simulink model "MIL4L3_SW6_V1_20220211"  (R2018b)
settings: Solver=FixedStepAuto  StartTime=0.0  StopTime=inf  FixedStep=0.001  RelTol=1e-3
PreLoadFcn:
  | A0_MILtest;
undefined symbols (not defined in the file or in its folder): Clb_ICADirect_LaneDisp_StateFive, Clb_ICADirect_LaneDisp_StateFour, Clb_ICADirect_LaneDisp_StateOne, Clb_ICADirect_LaneDisp_StateThree, Clb_ICADirect_LaneDisp_StateTwo, Clb_ICADirect_LaneDisp_StateZero, Clb_ICADirect_LaneDispSW, Clb_ICADirect_TrnLghtsCom_Switch, Clb_ICADirect_TrnLghtsCom_Value, Clb_ICADirect_TrnLghtsCrtl_Inhb, IMAP_Clb_ACU_Driver_Belt, IMAP_Clb_ACU_Driver_Belt_Over, IMAP_Clb_ACU_Passenger_Belt, IMAP_Clb_ACU_Passenger_Belt_Over, IMAP_Clb_ACU_RearLeft_Belt, IMAP_Clb_ACU_RearLeft_Belt_Over, IMAP_Clb_ACU_RearMiddle_Belt, IMAP_Clb_ACU_RearMiddle_Belt_Over, IMAP_Clb_ACU_RearRight_Belt, IMAP_Clb_ACU_RearRight_Belt_Over, IMAP_Clb_AEB_Switch, IMAP_Clb_AEB_Switch_Over, IMAP_Clb_ALC_TLC_Mode, IMAP_Clb_ALC_TLC_Mode_Over, IMAP_Clb_BCM_Battery_Voltage, IMAP_Clb_BCM_Battery_Voltage_Over, IMAP_Clb_BCM_BrakeLamp_State, IMAP_Clb_BCM_BrakeLamp_State_Over, IMAP_Clb_BCM_CHMSL_Status, IMAP_Clb_BCM_CHMSL_Status_Over, IMAP_Clb_BCM_Door_Lock_State, IMAP_Clb_BCM_Door_Lock_State_Over, IMAP_Clb_BCM_FrontWiper_State, IMAP_Clb_BCM_FrontWiper_State_Over, IMAP_Clb_BCM_FrontWiper_Switch, IMAP_Clb_BCM_FrontWiper_Switch_Over, IMAP_Clb_BCM_HazardLamp, IMAP_Clb_BCM_HazardLamp_Over, IMAP_Clb_BCM_HazardLamp_Switch, IMAP_Clb_BCM_HazardLamp_Switch_Over, IMAP_Clb_BCM_HighBeam_State, IMAP_Clb_BCM_HighBeam_State_Over, IMAP_Clb_BCM_Ignition_State, IMAP_Clb_BCM_Ignition_State_Over, IMAP_Clb_BCM_IHBC_Enabled, IMAP_Clb_BCM_IHBC_Enabled_Over, IMAP_Clb_BCM_Left_Light, IMAP_Clb_BCM_Left_Light_Over, IMAP_Clb_BCM_LeftTurn_Switch, IMAP_Clb_BCM_LeftTurn_Switch_Over, IMAP_Clb_BCM_LF_Door_State, IMAP_Clb_BCM_LF_Door_State_Over, IMAP_Clb_BCM_LowBeam_State, IMAP_Clb_BCM_LowBeam_State_Over, IMAP_Clb_BCM_LR_Door_State, IMAP_Clb_BCM_LR_Door_State_Over, IMAP_Clb_BCM_RF_Door_State, IMAP_Clb_BCM_RF_Door_State_Over, IMAP_Clb_BCM_Right_Light, IMAP_Clb_BCM_Right_Light_Over ... (+547)
libraries: CarMaker4SL x2153, simulink x292, dspstat3 x3, canmsglib x2, simulink_extras x1
(part 29 of 52)

== system MIL4L3_SW6_V1_20220211/CarMaker/VehicleControl/Data Inport/IMAP/Subsystem18/Subsystem5 ==
  In1 : Inport
  -1 : Constant
  -2 : Constant
  -3 : Constant  Value=13.515
  -4 : Constant
  0 : Constant
  1 : Constant  Value=15.604
  2 : Constant  Value=11.1
  3 : Constant  Value=6.986
  4 : Constant  Value=4.737
  5 : Constant  Value=3.311
  6 : Constant  Value=2.356
  Multiport Switch : MultiPortSwitch  DataPortOrder=Specify indices  Inputs=9  DataPortIndices={0,1,2,3,4,5,6,7,8,-1}  DataPortForDefault=Additional data port
  TCU_AGB_position : Outport
  wires:
  -4/1 -> Multiport Switch/12
  -3/1 -> Multiport Switch/11
  Multiport Switch/1 -> TCU_AGB_position/1  "TCU_AGB_position"
  -2/1 -> Multiport Switch/10
  6/1 -> Multiport Switch/8
  1/1 -> Multiport Switch/3
  5/1 -> Multiport Switch/7
  In1/1 -> Multiport Switch/1
  2/1 -> Multiport Switch/4
  0/1 -> Multiport Switch/2
  -1/1 -> Multiport Switch/9
  4/1 -> Multiport Switch/6
  3/1 -> Multiport Switch/5

== system MIL4L3_SW6_V1_20220211/CarMaker/VehicleControl/Data Inport/SDFA-L3/Subsystem4/Subsystem ==
  Constant4 : Constant  Value=0
  Digital Clock : DigitalClock  SampleTime=0.055
  Gain9 : Gain  Gain=100/5.5
  Switch : Switch  Threshold=65535
  Out1 : Outport
  wires:
  Digital Clock/1 -> Gain9/1
  Constant4/1 -> Switch/1
  Switch/1 -> Out1/1
  Gain9/1 -> Switch/2, Switch/3

== system MIL4L3_SW6_V1_20220211/CarMaker/VehicleControl/Data Inport/SDFA-L3/Subsystem4/Subsystem1 ==
  Constant4 : Constant  Value=0
  Digital Clock : DigitalClock  SampleTime=0.055
  Gain9 : Gain  Gain=100/5.5
  Switch : Switch  Threshold=65535
  Out1 : Outport
  wires:
  Gain9/1 -> Switch/3, Switch/2
  Switch/1 -> Out1/1
  Constant4/1 -> Switch/1
  Digital Clock/1 -> Gain9/1

== system MIL4L3_SW6_V1_20220211/CarMaker/VehicleControl/Data Inport/SDFA-L3/Subsystem4/Subsystem10 ==
  Constant4 : Constant  Value=0
  Digital Clock : DigitalClock  SampleTime=0.055
  Gain9 : Gain  Gain=100/5.5
  Switch : Switch  Threshold=65535
  Out1 : Outport
  wires:
  Digital Clock/1 -> Gain9/1
  Constant4/1 -> Switch/1
  Switch/1 -> Out1/1
  Gain9/1 -> Switch/2, Switch/3

== system MIL4L3_SW6_V1_20220211/CarMaker/VehicleControl/Data Inport/SDFA-L3/Subsystem4/Subsystem11 ==
  Constant4 : Constant  Value=0
  Digital Clock : DigitalClock  SampleTime=0.055
  Gain9 : Gain  Gain=100/5.5
  Switch : Switch  Threshold=65535
  Out1 : Outport
  wires:
  Gain9/1 -> Switch/3, Switch/2
  Switch/1 -> Out1/1
  Constant4/1 -> Switch/1
  Digital Clock/1 -> Gain9/1

== system MIL4L3_SW6_V1_20220211/CarMaker/VehicleControl/Data Inport/SDFA-L3/Subsystem4/Subsystem12 ==
  Constant4 : Constant  Value=0
  Digital Clock : DigitalClock  SampleTime=0.055
  Gain9 : Gain  Gain=100/5.5
  Switch : Switch  Threshold=65535
  Out1 : Outport
  wires:
  Digital Clock/1 -> Gain9/1
  Constant4/1 -> Switch/1
  Switch/1 -> Out1/1
  Gain9/1 -> Switch/2, Switch/3

== system MIL4L3_SW6_V1_20220211/CarMaker/VehicleControl/Data Inport/SDFA-L3/Subsystem4/Subsystem13 ==
  Constant4 : Constant  Value=0
  Digital Clock : DigitalClock  SampleTime=0.055
  Gain9 : Gain  Gain=100/5.5
  Switch : Switch  Threshold=65535
  Out1 : Outport
  wires:
  Gain9/1 -> Switch/3, Switch/2
  Switch/1 -> Out1/1
  Constant4/1 -> Switch/1
  Digital Clock/1 -> Gain9/1

== system MIL4L3_SW6_V1_20220211/CarMaker/VehicleControl/Data Inport/SDFA-L3/Subsystem4/Subsystem14 ==
  Constant4 : Constant  Value=0
  Digital Clock : DigitalClock  SampleTime=0.055
  Gain9 : Gain  Gain=100/5.5
  Switch : Switch  Threshold=65535
  Out1 : Outport
  wires:
  Gain9/1 -> Switch/3, Switch/2
  Switch/1 -> Out1/1
  Constant4/1 -> Switch/1
  Digital Clock/1 -> Gain9/1

== system MIL4L3_SW6_V1_20220211/CarMaker/VehicleControl/Data Inport/SDFA-L3/Subsystem4/Subsystem15 ==
  Constant4 : Constant  Value=0
  Digital Clock : DigitalClock  SampleTime=0.055
  Gain9 : Gain  Gain=100/5.5
  Switch : Switch  Threshold=65535
  Out1 : Outport
  wires:
  Digital Clock/1 -> Gain9/1
  Constant4/1 -> Switch/1
  Switch/1 -> Out1/1
  Gain9/1 -> Switch/2, Switch/3

== system MIL4L3_SW6_V1_20220211/CarMaker/VehicleControl/Data Inport/SDFA-L3/Subsystem4/Subsystem16 ==
  Constant4 : Constant  Value=0
  Digital Clock : DigitalClock  SampleTime=0.055
  Gain9 : Gain  Gain=100/5.5
  Switch : Switch  Threshold=65535
  Out1 : Outport
  wires:
  Gain9/1 -> Switch/3, Switch/2
  Switch/1 -> Out1/1
  Constant4/1 -> Switch/1
  Digital Clock/1 -> Gain9/1

== system MIL4L3_SW6_V1_20220211/CarMaker/VehicleControl/Data Inport/SDFA-L3/Subsystem4/Subsystem17 ==
  Constant4 : Constant  Value=0
  Digital Clock : DigitalClock  SampleTime=0.055
  Gain9 : Gain  Gain=100/5.5
  Switch : Switch  Threshold=65535
  Out1 : Outport
  wires:
  Digital Clock/1 -> Gain9/1
  Constant4/1 -> Switch/1
  Switch/1 -> Out1/1
  Gain9/1 -> Switch/2, Switch/3

== system MIL4L3_SW6_V1_20220211/CarMaker/VehicleControl/Data Inport/SDFA-L3/Subsystem4/Subsystem18 ==
  Constant4 : Constant  Value=0
  Digital Clock : DigitalClock  SampleTime=0.055
  Gain9 : Gain  Gain=100/5.5
  Switch : Switch  Threshold=65535
  Out1 : Outport
  wires:
  Digital Clock/1 -> Gain9/1
  Constant4/1 -> Switch/1
  Switch/1 -> Out1/1
  Gain9/1 -> Switch/2, Switch/3

== system MIL4L3_SW6_V1_20220211/CarMaker/VehicleControl/Data Inport/SDFA-L3/Subsystem4/Subsystem19 ==
  Constant4 : Constant  Value=0
  Digital Clock : DigitalClock  SampleTime=0.055
  Gain9 : Gain  Gain=100/5.5
  Switch : Switch  Threshold=65535
  Out1 : Outport
  wires:
  Gain9/1 -> Switch/3, Switch/2
  Switch/1 -> Out1/1
  Constant4/1 -> Switch/1
  Digital Clock/1 -> Gain9/1

== system MIL4L3_SW6_V1_20220211/CarMaker/VehicleControl/Data Inport/SDFA-L3/Subsystem4/Subsystem2 ==
  Constant4 : Constant  Value=0
  Digital Clock : DigitalClock  SampleTime=0.055
  Gain9 : Gain  Gain=100/5.5
  Switch : Switch  Threshold=65535
  Out1 : Outport
  wires:
  Gain9/1 -> Switch/3, Switch/2
  Switch/1 -> Out1/1
  Constant4/1 -> Switch/1
  Digital Clock/1 -> Gain9/1

== system MIL4L3_SW6_V1_20220211/CarMaker/VehicleControl/Data Inport/SDFA-L3/Subsystem4/Subsystem3 ==
  Constant4 : Constant  Value=0
  Digital Clock : DigitalClock  SampleTime=0.055
  Gain9 : Gain  Gain=100/5.5
  Switch : Switch  Threshold=65535
  Out1 : Outport
  wires:
  Digital Clock/1 -> Gain9/1
  Constant4/1 -> Switch/1
  Switch/1 -> Out1/1
  Gain9/1 -> Switch/2, Switch/3

== system MIL4L3_SW6_V1_20220211/CarMaker/VehicleControl/Data Inport/SDFA-L3/Subsystem4/Subsystem4 ==
  Constant4 : Constant  Value=0
  Digital Clock : DigitalClock  SampleTime=0.055
  Gain9 : Gain  Gain=100/5.5
  Switch : Switch  Threshold=65535
  Out1 : Outport
  wires:
  Gain9/1 -> Switch/3, Switch/2
  Switch/1 -> Out1/1
  Constant4/1 -> Switch/1
  Digital Clock/1 -> Gain9/1

== system MIL4L3_SW6_V1_20220211/CarMaker/VehicleControl/Data Inport/SDFA-L3/Subsystem4/Subsystem5 ==
  Constant4 : Constant  Value=0
  Digital Clock : DigitalClock  SampleTime=0.055
  Gain9 : Gain  Gain=100/5.5
  Switch : Switch  Threshold=65535
  Out1 : Outport
  wires:
  Digital Clock/1 -> Gain9/1
  Constant4/1 -> Switch/1
  Switch/1 -> Out1/1
  Gain9/1 -> Switch/2, Switch/3

== system MIL4L3_SW6_V1_20220211/CarMaker/VehicleControl/Data Inport/SDFA-L3/Subsystem4/Subsystem6 ==
  Constant4 : Constant  Value=0
  Digital Clock : DigitalClock  SampleTime=0.055
  Gain9 : Gain  Gain=100/5.5
  Switch : Switch  Threshold=65535
  Out1 : Outport
  wires:
  Digital Clock/1 -> Gain9/1
  Constant4/1 -> Switch/1
  Switch/1 -> Out1/1
  Gain9/1 -> Switch/2, Switch/3

== system MIL4L3_SW6_V1_20220211/CarMaker/VehicleControl/Data Inport/SDFA-L3/Subsystem4/Subsystem7 ==
  Constant4 : Constant  Value=0
  Digital Clock : DigitalClock  SampleTime=0.055
  Gain9 : Gain  Gain=100/5.5
  Switch : Switch  Threshold=65535
  Out1 : Outport
  wires:
  Gain9/1 -> Switch/3, Switch/2
  Switch/1 -> Out1/1
  Constant4/1 -> Switch/1
  Digital Clock/1 -> Gain9/1

== system MIL4L3_SW6_V1_20220211/CarMaker/VehicleControl/Data Inport/SDFA-L3/Subsystem4/Subsystem8 ==
  Constant4 : Constant  Value=0
  Digital Clock : DigitalClock  SampleTime=0.055
  Gain9 : Gain  Gain=100/5.5
  Switch : Switch  Threshold=65535
  Out1 : Outport
  wires:
  Gain9/1 -> Switch/3, Switch/2
  Switch/1 -> Out1/1
  Constant4/1 -> Switch/1
  Digital Clock/1 -> Gain9/1

== system MIL4L3_SW6_V1_20220211/CarMaker/VehicleControl/Data Inport/SDFA-L3/Subsystem4/Subsystem9 ==
  Constant4 : Constant  Value=0
  Digital Clock : DigitalClock  SampleTime=0.055
  Gain9 : Gain  Gain=100/5.5
  Switch : Switch  Threshold=65535
  Out1 : Outport
  wires:
  Digital Clock/1 -> Gain9/1
  Constant4/1 -> Switch/1
  Switch/1 -> Out1/1
  Gain9/1 -> Switch/2, Switch/3

== system MIL4L3_SW6_V1_20220211/CarMaker/VehicleControl/Data Inport/SDFA-L3/Subsystem40/Subsystem ==
  Compare To Constant : simulink/Logic and Bit Operations/Compare To Constant  relop=>=  const=1  OutDataTypeStr=boolean
  Compare To Constant1 : simulink/Logic and Bit Operations/Compare To Constant  relop=>  const=0  OutDataTypeStr=boolean
  Const tar_id5 : Constant  Value=0
  Data Type Conversion : DataTypeConversion
  Digital Clock : DigitalClock  SampleTime=0.06
  Logical Operator : Logic  AllPortsSameDT=off  OutDataTypeStr=boolean
  Read CM Dict1 : CarMaker4SL/Read CM Dict  xname=Sensor.Object.Radar.relvTgt.dtct  xsync=off
  Read CM Dict7 : CarMaker4SL/Read CM Dict  xname=User.IO.Out.NumberOfObj  xsync=off
  Switch15 : Switch  Criteria=u2 > Threshold
  Radar_timestamp : Outport
  wires:
  Logical Operator/1 -> Switch15/2  "<dtct>"
  Digital Clock/1 -> Data Type Conversion/1
  Data Type Conversion/1 -> Switch15/1
  Switch15/1 -> Radar_timestamp/1  "Radar_timestamp"
  Const tar_id5/1 -> Switch15/3
  Read CM Dict7/1 -> Compare To Constant/1
  Compare To Constant/1 -> Logical Operator/2
  Read CM Dict1/1 -> Compare To Constant1/1
  Compare To Constant1/1 -> Logical Operator/1

== system MIL4L3_SW6_V1_20220211/CarMaker/VehicleControl/Data Inport/SDFA-L3/Subsystem40/Subsystem1 ==
  Compare To Constant : simulink/Logic and Bit Operations/Compare To Constant  relop=>=  const=2  OutDataTypeStr=boolean
  Compare To Constant1 : simulink/Logic and Bit Operations/Compare To Constant  relop=>  const=0  OutDataTypeStr=boolean
  Const tar_id5 : Constant  Value=0
  Data Type Conversion : DataTypeConversion
  Digital Clock : DigitalClock  SampleTime=0.06
  Logical Operator : Logic  AllPortsSameDT=off  OutDataTypeStr=boolean
  Read CM Dict1 : CarMaker4SL/Read CM Dict  xname=Sensor.Object.Radar.relvTgt.dtct  xsync=off
  Read CM Dict7 : CarMaker4SL/Read CM Dict  xname=User.IO.Out.NumberOfObj  xsync=off
  Switch15 : Switch  Criteria=u2 > Threshold
  Radar_timestamp : Outport
  wires:
  Compare To Constant1/1 -> Logical Operator/1
  Read CM Dict1/1 -> Compare To Constant1/1
  Compare To Constant/1 -> Logical Operator/2
  Read CM Dict7/1 -> Compare To Constant/1
  Const tar_id5/1 -> Switch15/3
  Switch15/1 -> Radar_timestamp/1  "Radar_timestamp"
  Data Type Conversion/1 -> Switch15/1
  Digital Clock/1 -> Data Type Conversion/1
  Logical Operator/1 -> Switch15/2  "<dtct>"

== system MIL4L3_SW6_V1_20220211/CarMaker/VehicleControl/Data Inport/SDFA-L3/Subsystem40/Subsystem10 ==
  Constant4 : Constant  Value=0
  Digital Clock : DigitalClock  SampleTime=0.06
  Gain9 : Gain  Gain=50/3
  Switch : Switch  Threshold=65535
  Out1 : Outport
  wires:
  Digital Clock/1 -> Gain9/1
  Constant4/1 -> Switch/1
  Switch/1 -> Out1/1
  Gain9/1 -> Switch/2, Switch/3

== system MIL4L3_SW6_V1_20220211/CarMaker/VehicleControl/Data Inport/SDFA-L3/Subsystem40/Subsystem11 ==
  Constant4 : Constant  Value=0
  Digital Clock : DigitalClock  SampleTime=0.06
  Gain9 : Gain  Gain=50/3
  Switch : Switch  Threshold=65535
  Out1 : Outport
  wires:
  Gain9/1 -> Switch/3, Switch/2
  Switch/1 -> Out1/1
  Constant4/1 -> Switch/1
  Digital Clock/1 -> Gain9/1

== system MIL4L3_SW6_V1_20220211/CarMaker/VehicleControl/Data Inport/SDFA-L3/Subsystem40/Subsystem12 ==
  Constant4 : Constant  Value=0
  Digital Clock : DigitalClock  SampleTime=0.06
  Gain9 : Gain  Gain=50/3
  Switch : Switch  Threshold=65535
  Out1 : Outport
  wires:
  Gain9/1 -> Switch/3, Switch/2
  Switch/1 -> Out1/1
  Constant4/1 -> Switch/1
  Digital Clock/1 -> Gain9/1

== system MIL4L3_SW6_V1_20220211/CarMaker/VehicleControl/Data Inport/SDFA-L3/Subsystem40/Subsystem13 ==
  Constant4 : Constant  Value=0
  Digital Clock : DigitalClock  SampleTime=0.06
  Gain9 : Gain  Gain=50/3
  Switch : Switch  Threshold=65535
  Out1 : Outport
  wires:
  Digital Clock/1 -> Gain9/1
  Constant4/1 -> Switch/1
  Switch/1 -> Out1/1
  Gain9/1 -> Switch/2, Switch/3

== system MIL4L3_SW6_V1_20220211/CarMaker/VehicleControl/Data Inport/SDFA-L3/Subsystem40/Subsystem14 ==
  Constant4 : Constant  Value=0
  Digital Clock : DigitalClock  SampleTime=0.06
  Gain9 : Gain  Gain=50/3
  Switch : Switch  Threshold=65535
  Out1 : Outport
  wires:
  Gain9/1 -> Switch/3, Switch/2
  Switch/1 -> Out1/1
  Constant4/1 -> Switch/1
  Digital Clock/1 -> Gain9/1

== system MIL4L3_SW6_V1_20220211/CarMaker/VehicleControl/Data Inport/SDFA-L3/Subsystem40/Subsystem15 ==
  Constant4 : Constant  Value=0
  Digital Clock : DigitalClock  SampleTime=0.06
  Gain9 : Gain  Gain=50/3
  Switch : Switch  Threshold=65535
  Out1 : Outport
  wires:
  Digital Clock/1 -> Gain9/1
  Constant4/1 -> Switch/1
  Switch/1 -> Out1/1
  Gain9/1 -> Switch/2, Switch/3

== system MIL4L3_SW6_V1_20220211/CarMaker/VehicleControl/Data Inport/SDFA-L3/Subsystem40/Subsystem16 ==
  Constant4 : Constant  Value=0
  Digital Clock : DigitalClock  SampleTime=0.06
  Gain9 : Gain  Gain=50/3
  Switch : Switch  Threshold=65535
  Out1 : Outport
  wires:
  Digital Clock/1 -> Gain9/1
  Constant4/1 -> Switch/1
  Switch/1 -> Out1/1
  Gain9/1 -> Switch/2, Switch/3

== system MIL4L3_SW6_V1_20220211/CarMaker/VehicleControl/Data Inport/SDFA-L3/Subsystem40/Subsystem17 ==
  Constant4 : Constant  Value=0
  Digital Clock : DigitalClock  SampleTime=0.06
  Gain9 : Gain  Gain=50/3
  Switch : Switch  Threshold=65535
  Out1 : Outport
  wires:
  Gain9/1 -> Switch/3, Switch/2
  Switch/1 -> Out1/1
  Constant4/1 -> Switch/1
  Digital Clock/1 -> Gain9/1

== system MIL4L3_SW6_V1_20220211/CarMaker/VehicleControl/Data Inport/SDFA-L3/Subsystem40/Subsystem18 ==
  Constant4 : Constant  Value=0
  Digital Clock : DigitalClock  SampleTime=0.06
  Gain9 : Gain  Gain=50/3
  Switch : Switch  Threshold=65535
  Out1 : Outport
  wires:
  Digital Clock/1 -> Gain9/1
  Constant4/1 -> Switch/1
  Switch/1 -> Out1/1
  Gain9/1 -> Switch/2, Switch/3

== system MIL4L3_SW6_V1_20220211/CarMaker/VehicleControl/Data Inport/SDFA-L3/Subsystem40/Subsystem19 ==
  Constant4 : Constant  Value=0
  Digital Clock : DigitalClock  SampleTime=0.06
  Gain9 : Gain  Gain=50/3
  Switch : Switch  Threshold=65535
  Out1 : Outport
  wires:
  Gain9/1 -> Switch/3, Switch/2
  Switch/1 -> Out1/1
  Constant4/1 -> Switch/1
  Digital Clock/1 -> Gain9/1

== system MIL4L3_SW6_V1_20220211/CarMaker/VehicleControl/Data Inport/SDFA-L3/Subsystem40/Subsystem2 ==
  Compare To Constant : simulink/Logic and Bit Operations/Compare To Constant  relop=>=  const=3  OutDataTypeStr=boolean
  Compare To Constant1 : simulink/Logic and Bit Operations/Compare To Constant  relop=>  const=0  OutDataTypeStr=boolean
  Const tar_id5 : Constant  Value=0
  Data Type Conversion : DataTypeConversion
  Digital Clock : DigitalClock  SampleTime=0.06
  Logical Operator : Logic  AllPortsSameDT=off  OutDataTypeStr=boolean
  Read CM Dict1 : CarMaker4SL/Read CM Dict  xname=Sensor.Object.Radar.relvTgt.dtct  xsync=off
  Read CM Dict7 : CarMaker4SL/Read CM Dict  xname=User.IO.Out.NumberOfObj  xsync=off
  Switch15 : Switch  Criteria=u2 > Threshold
  Radar_timestamp : Outport
  wires:
  Logical Operator/1 -> Switch15/2  "<dtct>"
  Digital Clock/1 -> Data Type Conversion/1
  Data Type Conversion/1 -> Switch15/1
  Switch15/1 -> Radar_timestamp/1  "Radar_timestamp"
  Const tar_id5/1 -> Switch15/3
  Read CM Dict7/1 -> Compare To Constant/1
  Compare To Constant/1 -> Logical Operator/2
  Read CM Dict1/1 -> Compare To Constant1/1
  Compare To Constant1/1 -> Logical Operator/1

== system MIL4L3_SW6_V1_20220211/CarMaker/VehicleControl/Data Inport/SDFA-L3/Subsystem40/Subsystem20 ==
  Constant4 : Constant  Value=0
  Digital Clock : DigitalClock  SampleTime=0.06
  Gain9 : Gain  Gain=50/3
  Switch : Switch  Threshold=65535
  Out1 : Outport
  wires:
  Digital Clock/1 -> Gain9/1
  Constant4/1 -> Switch/1
  Switch/1 -> Out1/1
  Gain9/1 -> Switch/2, Switch/3

== system MIL4L3_SW6_V1_20220211/CarMaker/VehicleControl/Data Inport/SDFA-L3/Subsystem40/Subsystem21 ==
  Constant4 : Constant  Value=0
  Digital Clock : DigitalClock  SampleTime=0.06
  Gain9 : Gain  Gain=50/3
  Switch : Switch  Threshold=65535
  Out1 : Outport
  wires:
  Gain9/1 -> Switch/3, Switch/2
  Switch/1 -> Out1/1
  Constant4/1 -> Switch/1
  Digital Clock/1 -> Gain9/1

== system MIL4L3_SW6_V1_20220211/CarMaker/VehicleControl/Data Inport/SDFA-L3/Subsystem40/Subsystem22 ==
  Constant4 : Constant  Value=0
  Digital Clock : DigitalClock  SampleTime=0.06
  Gain9 : Gain  Gain=50/3
  Switch : Switch  Threshold=65535
  Out1 : Outport
  wires:
  Digital Clock/1 -> Gain9/1
  Constant4/1 -> Switch/1
  Switch/1 -> Out1/1
  Gain9/1 -> Switch/2, Switch/3

== system MIL4L3_SW6_V1_20220211/CarMaker/VehicleControl/Data Inport/SDFA-L3/Subsystem40/Subsystem23 ==
  Constant4 : Constant  Value=0
  Digital Clock : DigitalClock  SampleTime=0.06
  Gain9 : Gain  Gain=50/3
  Switch : Switch  Threshold=65535
  Out1 : Outport
  wires:
  Gain9/1 -> Switch/3, Switch/2
  Switch/1 -> Out1/1
  Constant4/1 -> Switch/1
  Digital Clock/1 -> Gain9/1

== system MIL4L3_SW6_V1_20220211/CarMaker/VehicleControl/Data Inport/SDFA-L3/Subsystem40/Subsystem24 ==
  Constant4 : Constant  Value=0
  Digital Clock : DigitalClock  SampleTime=0.06
  Gain9 : Gain  Gain=50/3
  Switch : Switch  Threshold=65535
  Out1 : Outport
  wires:
  Gain9/1 -> Switch/3, Switch/2
  Switch/1 -> Out1/1
  Constant4/1 -> Switch/1
  Digital Clock/1 -> Gain9/1

== system MIL4L3_SW6_V1_20220211/CarMaker/VehicleControl/Data Inport/SDFA-L3/Subsystem40/Subsystem25 ==
  Constant4 : Constant  Value=0
  Digital Clock : DigitalClock  SampleTime=0.06
  Gain9 : Gain  Gain=50/3
  Switch : Switch  Threshold=65535
  Out1 : Outport
  wires:
  Digital Clock/1 -> Gain9/1
  Constant4/1 -> Switch/1
  Switch/1 -> Out1/1
  Gain9/1 -> Switch/2, Switch/3

== system MIL4L3_SW6_V1_20220211/CarMaker/VehicleControl/Data Inport/SDFA-L3/Subsystem40/Subsystem26 ==
  Constant4 : Constant  Value=0
  Digital Clock : DigitalClock  SampleTime=0.06
  Gain9 : Gain  Gain=50/3
  Switch : Switch  Threshold=65535
  Out1 : Outport
  wires:
  Gain9/1 -> Switch/3, Switch/2
  Switch/1 -> Out1/1
  Constant4/1 -> Switch/1
  Digital Clock/1 -> Gain9/1

== system MIL4L3_SW6_V1_20220211/CarMaker/VehicleControl/Data Inport/SDFA-L3/Subsystem40/Subsystem27 ==
  Constant4 : Constant  Value=0
  Digital Clock : DigitalClock  SampleTime=0.06
  Gain9 : Gain  Gain=50/3
  Switch : Switch  Threshold=65535
  Out1 : Outport
  wires:
  Digital Clock/1 -> Gain9/1
  Constant4/1 -> Switch/1
  Switch/1 -> Out1/1
  Gain9/1 -> Switch/2, Switch/3

== system MIL4L3_SW6_V1_20220211/CarMaker/VehicleControl/Data Inport/SDFA-L3/Subsystem40/Subsystem3 ==
  Compare To Constant : simulink/Logic and Bit Operations/Compare To Constant  relop=>=  const=4  OutDataTypeStr=boolean
  Compare To Constant1 : simulink/Logic and Bit Operations/Compare To Constant  relop=>  const=0  OutDataTypeStr=boolean
  Const tar_id5 : Constant  Value=0
  Data Type Conversion : DataTypeConversion
  Digital Clock : DigitalClock  SampleTime=0.06
  Logical Operator : Logic  AllPortsSameDT=off  OutDataTypeStr=boolean
  Read CM Dict1 : CarMaker4SL/Read CM Dict  xname=Sensor.Object.Radar.relvTgt.dtct  xsync=off
  Read CM Dict7 : CarMaker4SL/Read CM Dict  xname=User.IO.Out.NumberOfObj  xsync=off
  Switch15 : Switch  Criteria=u2 > Threshold
  Radar_timestamp : Outport
  wires:
  Compare To Constant1/1 -> Logical Operator/1
  Read CM Dict1/1 -> Compare To Constant1/1
  Compare To Constant/1 -> Logical Operator/2
  Read CM Dict7/1 -> Compare To Constant/1
  Const tar_id5/1 -> Switch15/3
  Switch15/1 -> Radar_timestamp/1  "Radar_timestamp"
  Data Type Conversion/1 -> Switch15/1
  Digital Clock/1 -> Data Type Conversion/1
  Logical Operator/1 -> Switch15/2  "<dtct>"

== system MIL4L3_SW6_V1_20220211/CarMaker/VehicleControl/Data Inport/SDFA-L3/Subsystem40/Subsystem4 ==
  Constant4 : Constant  Value=0
  Digital Clock : DigitalClock  SampleTime=0.06
  Gain9 : Gain  Gain=50/3
  Switch : Switch  Threshold=65535
  Out1 : Outport
  wires:
  Digital Clock/1 -> Gain9/1
  Constant4/1 -> Switch/1
  Switch/1 -> Out1/1
  Gain9/1 -> Switch/2, Switch/3

== system MIL4L3_SW6_V1_20220211/CarMaker/VehicleControl/Data Inport/SDFA-L3/Subsystem40/Subsystem5 ==
  Constant4 : Constant  Value=0
  Digital Clock : DigitalClock  SampleTime=0.06
  Gain9 : Gain  Gain=50/3
  Switch : Switch  Threshold=65535
  Out1 : Outport
  wires:
  Gain9/1 -> Switch/3, Switch/2
  Switch/1 -> Out1/1
  Constant4/1 -> Switch/1
  Digital Clock/1 -> Gain9/1

== system MIL4L3_SW6_V1_20220211/CarMaker/VehicleControl/Data Inport/SDFA-L3/Subsystem40/Subsystem6 ==
  Constant4 : Constant  Value=0
  Digital Clock : DigitalClock  SampleTime=0.06
  Gain9 : Gain  Gain=50/3
  Switch : Switch  Threshold=65535
  Out1 : Outport
  wires:
  Gain9/1 -> Switch/3, Switch/2
  Switch/1 -> Out1/1
  Constant4/1 -> Switch/1
  Digital Clock/1 -> Gain9/1

== system MIL4L3_SW6_V1_20220211/CarMaker/VehicleControl/Data Inport/SDFA-L3/Subsystem40/Subsystem7 ==
  Constant4 : Constant  Value=0
  Digital Clock : DigitalClock  SampleTime=0.06
  Gain9 : Gain  Gain=50/3
  Switch : Switch  Threshold=65535
  Out1 : Outport
  wires:
  Digital Clock/1 -> Gain9/1
  Constant4/1 -> Switch/1
  Switch/1 -> Out1/1
  Gain9/1 -> Switch/2, Switch/3

== system MIL4L3_SW6_V1_20220211/CarMaker/VehicleControl/Data Inport/SDFA-L3/Subsystem40/Subsystem8 ==
  Constant4 : Constant  Value=0
  Digital Clock : DigitalClock  SampleTime=0.06
  Gain9 : Gain  Gain=50/3
  Switch : Switch  Threshold=65535
  Out1 : Outport
  wires:
  Gain9/1 -> Switch/3, Switch/2
  Switch/1 -> Out1/1
  Constant4/1 -> Switch/1
  Digital Clock/1 -> Gain9/1

== system MIL4L3_SW6_V1_20220211/CarMaker/VehicleControl/Data Inport/SDFA-L3/Subsystem40/Subsystem9 ==
  Constant4 : Constant  Value=0
  Digital Clock : DigitalClock  SampleTime=0.06
  Gain9 : Gain  Gain=50/3
  Switch : Switch  Threshold=65535
  Out1 : Outport
  wires:
  Digital Clock/1 -> Gain9/1
  Constant4/1 -> Switch/1
  Switch/1 -> Out1/1
  Gain9/1 -> Switch/2, Switch/3

== system MIL4L3_SW6_V1_20220211/CarMaker/VehicleControl/Data Inport/SDFA-L3/Subsystem41/Subsystem ==
  Const tar_id5 : Constant  Value=0
  Data Type Conversion : DataTypeConversion
  Digital Clock : DigitalClock  SampleTime=0.06
  Read CM Dict7 : CarMaker4SL/Read CM Dict  xname=User.IO.Out.IFC_obj01_Timestamp  xsync=off
  Switch15 : Switch  Criteria=u2 > Threshold
  camera_timestamp : Outport
  wires:
  Digital Clock/1 -> Data Type Conversion/1
  Data Type Conversion/1 -> Switch15/1
  Switch15/1 -> camera_timestamp/1  "camera_timestamp"
  Const tar_id5/1 -> Switch15/3
  Read CM Dict7/1 -> Switch15/2

== system MIL4L3_SW6_V1_20220211/CarMaker/VehicleControl/Data Inport/SDFA-L3/Subsystem41/Subsystem1 ==
  Const tar_id5 : Constant  Value=0
  Data Type Conversion : DataTypeConversion
  Digital Clock : DigitalClock  SampleTime=0.06
  Read CM Dict7 : CarMaker4SL/Read CM Dict  xname=User.IO.Out.IFC_obj02_Timestamp  xsync=off
  Switch15 : Switch  Criteria=u2 > Threshold
  camera_timestamp : Outport
  wires:
  Digital Clock/1 -> Data Type Conversion/1
  Const tar_id5/1 -> Switch15/3
  Switch15/1 -> camera_timestamp/1  "camera_timestamp"
  Data Type Conversion/1 -> Switch15/1
  Read CM Dict7/1 -> Switch15/2

== system MIL4L3_SW6_V1_20220211/CarMaker/VehicleControl/Data Inport/SDFA-L3/Subsystem41/Subsystem2 ==
  Const tar_id5 : Constant  Value=0
  Data Type Conversion : DataTypeConversion
  Digital Clock : DigitalClock  SampleTime=0.06
  Read CM Dict7 : CarMaker4SL/Read CM Dict  xname=User.IO.Out.IFC_obj03_Timestamp  xsync=off
  Switch15 : Switch  Criteria=u2 > Threshold
  camera_timestamp : Outport
  wires:
  Digital Clock/1 -> Data Type Conversion/1
  Const tar_id5/1 -> Switch15/3
  Switch15/1 -> camera_timestamp/1  "camera_timestamp"
  Data Type Conversion/1 -> Switch15/1
  Read CM Dict7/1 -> Switch15/2

== system MIL4L3_SW6_V1_20220211/CarMaker/VehicleControl/Data Inport/SDFA-L3/Subsystem41/Subsystem3 ==
  Const tar_id5 : Constant  Value=0
  Data Type Conversion : DataTypeConversion
  Digital Clock : DigitalClock  SampleTime=0.06
  Read CM Dict7 : CarMaker4SL/Read CM Dict  xname=User.IO.Out.IFC_obj04_Timestamp  xsync=off
  Switch15 : Switch  Criteria=u2 > Threshold
  camera_timestamp : Outport
  wires:
  Digital Clock/1 -> Data Type Conversion/1
  Const tar_id5/1 -> Switch15/3
  Switch15/1 -> camera_timestamp/1  "camera_timestamp"
  Data Type Conversion/1 -> Switch15/1
  Read CM Dict7/1 -> Switch15/2

== system MIL4L3_SW6_V1_20220211/CarMaker/VehicleControl/Function/ICA/EPS Position Control Enable Management (EPSPCEM)_KDK1/EPS_Ctr_Disable ==
  stEPSCtlState : Inport
  Action Port : ActionPort  InitializeStates=reset  ActionType=else
  MATLAB Function : MATLAB Function  TreatAsAtomicUnit=on
  stEPSCtlCMD : Outport
  wires:
  MATLAB Function/1(stEPSCtlCMD) -> stEPSCtlCMD/1
  stEPSCtlState/1 -> MATLAB Function/1(stEPSCtlState)

== system MIL4L3_SW6_V1_20220211/CarMaker/VehicleControl/Function/ICA/EPS Position Control Enable Management (EPSPCEM)_KDK1/EPS_Ctr_Enable ==
  stEPSCtlState : Inport
  Action Port : ActionPort  InitializeStates=reset  ActionType=then
  MATLAB Function : MATLAB Function  TreatAsAtomicUnit=on
  stEPSCtlCMD : Outport
  wires:
  stEPSCtlState/1 -> MATLAB Function/1(stEPSCtlState)
  MATLAB Function/1(stEPSCtlCMD) -> stEPSCtlCMD/1

== system MIL4L3_SW6_V1_20220211/CarMaker/VehicleControl/Function/ICA_ALC/EPS Position Control Enable Management (EPSPCEM)_KDK1/EPS_Ctr_Disable ==
  stEPSCtlState : Inport
  Action Port : ActionPort  InitializeStates=reset  ActionType=else
  MATLAB Function : MATLAB Function  TreatAsAtomicUnit=on
  stEPSCtlCMD : Outport
  wires:
  stEPSCtlState/1 -> MATLAB Function/1(stEPSCtlState)
  MATLAB Function/1(stEPSCtlCMD) -> stEPSCtlCMD/1

== system MIL4L3_SW6_V1_20220211/CarMaker/VehicleControl/Function/ICA_ALC/EPS Position Control Enable Management (EPSPCEM)_KDK1/EPS_Ctr_Enable ==
  stEPSCtlState : Inport
  Action Port : ActionPort  InitializeStates=reset  ActionType=then
  MATLAB Function : MATLAB Function  TreatAsAtomicUnit=on
  stEPSCtlCMD : Outport
  wires:
  MATLAB Function/1(stEPSCtlCMD) -> stEPSCtlCMD/1
  stEPSCtlState/1 -> MATLAB Function/1(stEPSCtlState)

== system MIL4L3_SW6_V1_20220211/CarMaker/VehicleControl/Function/LKA/LKAS1/LL ==
  bsInInfo : Inport
  bsLLClb : Inport  Port=2
  Bus Selector : BusSelector  OutputSignals=bsMP5Info.LKA_Mode
  Bus Selector1 : BusSelector  OutputSignals=bsLaneInfo.bsR0Info.R0_Q,bsLaneInfo.bsL0Info.L0_Q
  Bus Selector2 : BusSelector  OutputSignals=bsEPSInfo
  Bus Selector3 : BusSelector  OutputSignals=LKA_State,LDW_State
  Bus Selector4 : BusSelector  OutputSignals=bsLaneInfo.Fusion_AdditionalInf.Carema_Status
  Bus Selector5 : BusSelector  OutputSignals=bsMP5Info.LKA_Mode
  Fault_Diagnostic : Subsystem
  Ground1 : Ground
  Human Machine Interface (HMI) : Subsystem
  LL Inputs Mapping : Subsystem
  LLOn : Subsystem
  LLOut : Subsystem
  Terminator : Terminator
  Version : Constant  Value=220224  OutMin=20410  OutMax=220630  OutDataTypeStr=single
  LL_bsLLOut : Outport
      settings: AttributesFormatString=Disable Action: %<OutputWhenDisabled>
  tag scope: LLMon=global
  wires:
  [LLOn_bsLDWWarnInfo] -> Human Machine Interface (HMI)/4(HMI_LDWWarn)
  Bus Selector2/1 -> Human Machine Interface (HMI)/7(HMI_EPSInfo)  "<bsEPSInfo>"
  Bus Selector1/2 -> Human Machine Interface (HMI)/6(HMI_L0_Quality)  "<L0_Q>"
  Bus Selector1/1 -> Human Machine Interface (HMI)/5(HMI_R0_Quality)  "<R0_Q>"
  Bus Selector5/1 -> Human Machine Interface (HMI)/1(HMI_stDACmode)  "<LKA_Mode>"
  [LLOn_bsLLState] -> Bus Selector3/1
  Bus Selector4/1 -> Human Machine Interface (HMI)/9(HMI_Front_Camera_Blocked)  "<Carema_Status>"
  Ground1/1 -> Human Machine Interface (HMI)/8(HMI_camera_common_fault)
  Bus Selector3/1 -> Human Machine Interface (HMI)/2(HMI_LKA_STATE)  "<LKA_State>"
  Bus Selector3/2 -> Human Machine Interface (HMI)/3(HMI_LDW_STATE)  "<LDW_State>"
  [bsInfo] -> Bus Selector5/1, Bus Selector1/1, Bus Selector2/1, Bus Selector4/1
  [LLOn_phiSWACmd] -> LLOut/2(LLOut_phiSWACmd)
  [bsInfo] -> LLOut/5(LLOut_bsInfo)
  [LLOn_M] -> LLOut/4(LLOut_M)
  [LLOn_bsLLState] -> LLOut/1(LLOut_bsLLState)
  LLOut/1(LL_bsLLOut) -> LL_bsLLOut/1
  [HMI_bsLLHMI] -> LLOut/3(LLOut_bsLLHMI)
  Bus Selector/1 -> LLOn/Enable  "<LKA_Mode>"
  bsInInfo/1 -> [bsInInfo]
  Human Machine Interface (HMI)/1(HMI_LDWLKA) -> [HMI_bsLLHMI]  "bsLLHMI"
  Version/1 -> Terminator/1  "ob_LKA_Version"
  LLOn/2(LDW_Flag) -> [LLOn_bsLDWWarnInfo]
  bsLLClb/1 -> [bsLLClb]
  LLOn/1(bsLLState) -> [LLOn_bsLLState]
  LLOn/3(phiSWACmd) -> [LLOn_phiSWACmd]
  LLOn/4(M) -> [LLOn_M]
  LLOn/5(LLMon) -> [LLMon]
  Fault_Diagnostic/1(bsSignalFault) -> [bsSignalFault]
  [bsInInfo] -> Fault_Diagnostic/1(bsInInfo)
  LL Inputs Mapping/1(bsInfo) -> [bsInfo]
  [bsInInfo] -> LL Inputs Mapping/1(bsInInfo)
  [bsInfo] -> Bus Selector/1, LLOn/1(bsInInfo)
  [bsLLClb] -> LLOn/2(bsLLClb)
  [bsSignalFault] -> LLOn/3(bsSignalFault)
  [bsLLClb] -> Human Machine Interface (HMI)/10(HMI_bsLLClb)
  [bsLLClb] -> LL Inputs Mapping/2(bsLLClb)

== system MIL4L3_SW6_V1_20220211/CarMaker/VehicleControl/Function/LKA/LKAS1/LLClb ==
  Bus Creator : BusCreator  Inputs=4
  ConstantClb : Subsystem
  LDWClb : Subsystem
  LKAClb : Subsystem
  LLSMConClb : Subsystem
  LLClb_bsLLClb : Outport
  wires:
  ConstantClb/1(ConstantClb) -> Bus Creator/4  "bsConstantClb"
  LLSMConClb/1(LLSMConClb) -> Bus Creator/1  "bsLLSMConClb"
  Bus Creator/1 -> LLClb_bsLLClb/1  "bsLLClb"
  LDWClb/1(LDWClb) -> Bus Creator/2  "bsLDWClb"
  LKAClb/1(LKAClb) -> Bus Creator/3  "bsLKAClb"

== system MIL4L3_SW6_V1_20220211/CarMaker/VehicleControl/Function/LKA/LKAS1/Output ==
  bsLLOut : Inport
  Bus Selector : BusSelector  OutputSignals=Vehicle_Lane_Display,LDW_Status_Display,LKA_Status_Display,LDW_Flag,Hands_Off_Warning,LKA_Action_Indication,HMI_Popup_Status,LKA_Torque_Req,LKA_TorqueReq_Value,EPS_State_Ctl,LKA_SWA_Control,EPS_Factor_Control,EPS_LKA_Control
  Cast To Single{1..9,12} (10 alike) : DataTypeConversion  OutDataTypeStr=UInt8
  Cast To Single10 : DataTypeConversion  OutDataTypeStr=T_M_Nm_Float32
  Cast To Single11 : DataTypeConversion  OutDataTypeStr=T_M_Nm_Float32
  Cast To Single13 : DataTypeConversion  OutDataTypeStr=T_M_Nm_Float32
  Vehicle_Lane_Display : Outport
  LDW_Status_Display : Outport  Port=2
  LKA_Status_Display : Outport  Port=3
  LDW_Flag : Outport  Port=4
  Hands_Off_Warning : Outport  Port=5
  LKA_Action_Indication : Outport  Port=6
  HMI_Popup_Status : Outport  Port=7
  LKA_TorqueReq : Outport  Port=8
  LKA_TorqueReq_Value : Outport  Port=9
  EPS_State_Control : Outport  Port=10
  LKA_SWA_Control : Outport  Port=11
  EPS_Factor_Control : Outport  Port=12
  EPS_LKA_Control : Outport  Port=13
  wires:
  Cast To Single1/1 -> Vehicle_Lane_Display/1  "Vehicle_Lane_Display"
  Cast To Single2/1 -> LDW_Status_Display/1  "LDW_Status_Display"
  Cast To Single3/1 -> LKA_Status_Display/1  "LKA_Status_Display"
  Cast To Single4/1 -> LDW_Flag/1  "LDW_Flag"
  Cast To Single5/1 -> Hands_Off_Warning/1  "Hands_Off_Warning"
  Cast To Single6/1 -> LKA_Action_Indication/1  "LKA_Action_Indication"
  Cast To Single7/1 -> HMI_Popup_Status/1  "HMI_Popup_Status"
  Cast To Single8/1 -> EPS_State_Control/1  "EPS_State_Control"
  Cast To Single9/1 -> EPS_LKA_Control/1  "EPS_LKA_Control"
  Cast To Single10/1 -> EPS_Factor_Control/1  "EPS_Factor_Control"
  Cast To Single11/1 -> LKA_SWA_Control/1  "LKA_SWA_Control"
  Cast To Single12/1 -> LKA_TorqueReq/1  "LKA_TorqueReq"
  Cast To Single13/1 -> LKA_TorqueReq_Value/1  "LKA_TorqueReq_Value"
  Bus Selector/9 -> Cast To Single13/1  "<LKA_TorqueReq_Value>"
  Bus Selector/8 -> Cast To Single12/1  "<LKA_Torque_Req>"
  Bus Selector/4 -> Cast To Single4/1  "<LDW_Flag>"
  Bus Selector/3 -> Cast To Single3/1  "<LKA_Status_Display>"
  Bus Selector/12 -> Cast To Single10/1  "<EPS_Factor_Control>"
  Bus Selector/6 -> Cast To Single6/1  "<LKA_Action_Indication>"
  Bus Selector/7 -> Cast To Single7/1  "<HMI_Popup_Status>"
  Bus Selector/5 -> Cast To Single5/1  "<Hands_Off_Warning>"
  Bus Selector/1 -> Cast To Single1/1  "<Vehicle_Lane_Display>"
  Bus Selector/10 -> Cast To Single8/1  "<EPS_State_Ctl>"
  bsLLOut/1 -> Bus Selector/1  "bsLLOutput"
  Bus Selector/11 -> Cast To Single11/1  "<LKA_SWA_Control>"
  Bus Selector/13 -> Cast To Single9/1  "<EPS_LKA_Control>"
  Bus Selector/2 -> Cast To Single2/1  "<LDW_Status_Display>"

== system MIL4L3_SW6_V1_20220211/CarMaker/VehicleControl/Function/LKA/LKAS1/SignalBusCreator ==
  LkaFcnConf : Inport
  LKA_Main_Switch : Inport  Port=2
  LKA_Mode : Inport  Port=3
  LDW_Warn_Mode : Inport  Port=4
  APA_AutoPark_WorkSt : Inport  Port=5
  MP5_Work_State : Inport  Port=6
  EPS_LKA_State : Inport  Port=7
  EPS_SW_Trq : Inport  Port=8
  EPS_Trq_State : Inport  Port=9
  SAS_Clb_State : Inport  Port=10
  SAS_Trim_State : Inport  Port=11
  SWS_Failure_Status : Inport  Port=12
  EPS_TrqLim_State : Inport  Port=13
  EPS_LKA_Current : Inport  Port=14
  EPS_SWHold_State : Inport  Port=15
  EPS_Driver_Override : Inport  Port=16
  EPS_ESA_State : Inport  Port=17
  EPS_SteeringAngle_Flag : Inport  Port=18
  EPS_SteeringAngle : Inport  Port=19
  SW_Angle : Inport  Port=20
  SW_Angle_Speed : Inport  Port=21
  ESC_LatAcc : Inport  Port=22
  ESC_LatAcc_Valid : Inport  Port=23
  ESC_YawRate : Inport  Port=24
  ESC_YawRate_Valid : Inport  Port=25
  ESC_UnYawRate : Inport  Port=26
  ESC_VehSpd : Inport  Port=27
  ESC_LonAcc : Inport  Port=28
  ESC_LonAcc_Valid : Inport  Port=29
  ESC_Brake_Press : Inport  Port=30
  ESC_VehSpd_Valid : Inport  Port=31
  BCM_Double_Light : Inport  Port=32
  BCM_Left_Light : Inport  Port=33
  BCM_Right_Light : Inport  Port=34
  BCM_LeftTurn_Switch : Inport  Port=35
  BCM_RightTurn_Switch : Inport  Port=36
  BCM_Double_Light_Switch : Inport  Port=37
  AccPedal_Pos : Inport  Port=38
  TCU_ActualGear : Inport  Port=39
  TCU_Available : Inport  Port=40
  ADIAve_g_ASWFaultStatus : Inport  Port=41
  ADIAve_g_BSWFaultStatus : Inport  Port=42
  ADIAve_d_FuncFaultStatus : Inport  Port=43
  Camera_Status : Inport  Port=44
  Sensor_Status : Inport  Port=45
  Fusion_Status : Inport  Port=46
  L0_C0 : Inport  Port=47
  L0_C1 : Inport  Port=48
  L0_C2 : Inport  Port=49
  L0_C3 : Inport  Port=50
  L0_VR : Inport  Port=51
  L0_Q : Inport  Port=52
  L0_Type : Inport  Port=53
  L0_W : Inport  Port=54
  R0_C0 : Inport  Port=55
  R0_C1 : Inport  Port=56
  R0_C2 : Inport  Port=57
  R0_C3 : Inport  Port=58
  R0_VR : Inport  Port=59
  R0_Q : Inport  Port=60
  R0_Type : Inport  Port=61
  R0_W : Inport  Port=62
  L1_C0 : Inport  Port=63
  L1_C1 : Inport  Port=64
  L1_C2 : Inport  Port=65
  L1_C3 : Inport  Port=66
  L1_VR : Inport  Port=67
  L1_Q : Inport  Port=68
  L1_Type : Inport  Port=69
  L1_W : Inport  Port=70
  R1_C0 : Inport  Port=71
  R1_C1 : Inport  Port=72
  R1_C2 : Inport  Port=73
  R1_C3 : Inport  Port=74
  R1_VR : Inport  Port=75
  R1_Q : Inport  Port=76
  R1_Type : Inport  Port=77
  R1_W : Inport  Port=78
  Bus Creator : BusCreator  Inputs=6
  Bus Creator1 : BusCreator  Inputs=6
  Bus Creator11 : BusCreator  Inputs=3
  Bus Creator{7..8,15..16} (4 alike) : BusCreator  Inputs=8
  Bus Creator2 : BusCreator  Inputs=11
  Bus Creator23 : BusCreator  Inputs=5
  Bus Creator3 : BusCreator  Inputs=4
  Bus Creator4 : BusCreator  Inputs=3
  Bus Creator5 : BusCreator  Inputs=9
  Bus Creator9 : BusCreator  Inputs=10
  DTC_Indicator : Subsystem
  Gain : Gain
  Gain1 : Gain
  Gain2 : Gain
  State : Subsystem
  Terminator : Terminator
  Terminator1 : Terminator
  Terminator2 : Terminator
  bsInInfo : Outport
  wires:
  Bus Creator9/1 -> [bsVehMovInfo]  "bsVehMovInfo"
  Bus Creator3/1 -> [bsSWAInfo]  "bsSWAInfo"
  Bus Creator1/1 -> [bsBCMInfo]  "bsBESState"
  Bus Creator2/1 -> [bsEPSInfo]  "bsEPSInfo"
  Bus Creator/1 -> [bsMP5Info]  "bsMP5Info"
  [bsLaneInfo] -> Bus Creator5/2  "bsLaneInfo"
  [bsEPSInfo] -> Bus Creator5/3  "bsEPSInfo"
  [bsVehMovInfo] -> Bus Creator5/4  "bsVehMovInfo"
  [bsSWAInfo] -> Bus Creator5/5  "bsSWAInfo"
  [bsBCMInfo] -> Bus Creator5/6  "bsBCMInfo"
  [bsPTState] -> Bus Creator5/7  "bsPTState"
  [bsMP5Info] -> Bus Creator5/1  "bsMP5Info"
  [bsStateInfo] -> Bus Creator5/8  "State"
  [bsDTC_Indicator] -> Bus Creator5/9  "DTC_Indicator"
  Bus Creator4/1 -> [bsPTState]  "bsPTState"
  Bus Creator7/1 -> [bsFusR0Info]  "bsFusR0Info"
  Bus Creator16/1 -> [bsFusL1Info]  "bsFusL1Info"
  Bus Creator15/1 -> [bsFusR1Info]  "bsFusR1Info"
  Bus Creator8/1 -> [bsFusL0Info]  "bsFusL0Info"
  [bsFusL0Info] -> Bus Creator23/1  "bsFusL0Info"
  [bsFusR0Info] -> Bus Creator23/2  "bsFusR0Info"
  [bsFusL1Info] -> Bus Creator23/3  "bsFusL1Info"
  [bsFusR1Info] -> Bus Creator23/4  "bsFusR1Info"
  Bus Creator23/1 -> [bsLaneInfo]  "bsLaneInfo"
  [Fusion_AdditionalInf] -> Bus Creator23/5  "Fusion_AdditionalInf"
  DTC_Indicator/1(bsDTC_Indicator) -> [bsDTC_Indicator]  "DTC_Indicator"
  State/1(bsStateInfo) -> [bsStateInfo]  "State"
  Bus Creator5/1 -> bsInInfo/1  "bsInInfo"
  AccPedal_Pos/1 -> Bus Creator4/1  "AccPedal_Pos"
  TCU_ActualGear/1 -> Bus Creator4/2  "TCU_ActualGear"
  BCM_Double_Light/1 -> Bus Creator1/1  "BCM_Double_Light"
  BCM_Left_Light/1 -> Bus Creator1/2  "BCM_Left_Light"
  BCM_Right_Light/1 -> Bus Creator1/3  "BCM_Right_Light"
  SW_Angle/1 -> Bus Creator3/3  "SW_Angle"
  SW_Angle_Speed/1 -> Bus Creator3/4  "SW_Angle_Speed"
  SWS_Failure_Status/1 -> Bus Creator2/6  "SWS_Failure_Status"
  ESC_LatAcc/1 -> Bus Creator9/1  "ESC_LatAcc"
  ESC_LatAcc_Valid/1 -> Bus Creator9/2  "ESC_LatAcc_Valid"
  ESC_YawRate/1 -> Bus Creator9/3  "ESC_YawRate"
  ESC_YawRate_Valid/1 -> Bus Creator9/4  "ESC_YawRate_Valid"
  ESC_UnYawRate/1 -> Bus Creator9/5  "ESC_UnYawRate"
  ESC_VehSpd/1 -> Bus Creator9/6  "ESC_VehSpd"
  ESC_LonAcc/1 -> Bus Creator9/7  "ESC_LonAcc"
  ESC_LonAcc_Valid/1 -> Bus Creator9/8  "ESC_LonAcc_Valid"
  ESC_Brake_Press/1 -> Bus Creator9/9  "ESC_Brake_Press"
  ESC_VehSpd_Valid/1 -> Bus Creator9/10  "ESC_VehSpd_Valid"
  EPS_LKA_State/1 -> Bus Creator2/1  "EPS_LKA_State"
  EPS_SW_Trq/1 -> Bus Creator2/2  "EPS_SW_Trq"
  EPS_Trq_State/1 -> Bus Creator2/3  "EPS_Trq_State"
  SAS_Clb_State/1 -> Bus Creator2/4  "SAS_Clb_State"
  SAS_Trim_State/1 -> Bus Creator2/5  "SAS_Trim_State"
  EPS_TrqLim_State/1 -> Bus Creator2/7  "EPS_TrqLim_State"
  EPS_LKA_Current/1 -> Bus Creator2/8  "EPS_LKA_Current"
  EPS_SWHold_State/1 -> Bus Creator2/9  "EPS_SWHold_State"
  LKA_Main_Switch/1 -> Bus Creator/2  "LKA_Main_Switch"
  LKA_Mode/1 -> Bus Creator/3  "LKA_Mode"
  L0_C0/1 -> Bus Creator8/1  "L0_C0"
  L0_C1/1 -> Bus Creator8/2  "L0_C1"
  L0_C2/1 -> Bus Creator8/3  "L0_C2"
  L0_C3/1 -> Bus Creator8/4  "L0_C3"
  L0_VR/1 -> Bus Creator8/5  "L0_VR"
  L0_Q/1 -> Bus Creator8/6  "L0_Q"
  L0_Type/1 -> Bus Creator8/7  "L0_Type"
  L0_W/1 -> Bus Creator8/8  "L0_W"
  R0_C0/1 -> Bus Creator7/1  "R0_C0"
  R0_C1/1 -> Bus Creator7/2  "R0_C1"
  R0_C2/1 -> Bus Creator7/3  "R0_C2"
  R0_C3/1 -> Bus Creator7/4  "R0_C3"
  R0_VR/1 -> Bus Creator7/5  "R0_VR"
  R0_Q/1 -> Bus Creator7/6  "R0_Q"
  R0_Type/1 -> Bus Creator7/7  "R0_Type"
  R0_W/1 -> Bus Creator7/8  "R0_W"
  L1_C0/1 -> Bus Creator16/1  "L1_C0"
  L1_C1/1 -> Bus Creator16/2  "L1_C1"
  L1_C2/1 -> Bus Creator16/3  "L1_C2"
  L1_C3/1 -> Bus Creator16/4  "L1_C3"
  L1_VR/1 -> Bus Creator16/5  "L1_VR"
  L1_Q/1 -> Bus Creator16/6  "L1_Q"
  L1_Type/1 -> Bus Creator16/7  "L1_Type"
  L1_W/1 -> Bus Creator16/8  "L1_W"
  R1_C0/1 -> Bus Creator15/1  "R1_C0"
  R1_C1/1 -> Bus Creator15/2  "R1_C1"
  R1_C2/1 -> Bus Creator15/3  "R1_C2"
  R1_C3/1 -> Bus Creator15/4  "R1_C3"
  R1_VR/1 -> Bus Creator15/5  "R1_VR"
  R1_Q/1 -> Bus Creator15/6  "R1_Q"
  R1_Type/1 -> Bus Creator15/7  "R1_Type"
  R1_W/1 -> Bus Creator15/8  "R1_W"
  TCU_Available/1 -> Bus Creator4/3  "TCU_Available"
  BCM_LeftTurn_Switch/1 -> Bus Creator1/4  "BCM_LeftTurn_Switch"
  BCM_RightTurn_Switch/1 -> Bus Creator1/5  "BCM_RightTurn_Switch"
  EPS_SteeringAngle_Flag/1 -> Bus Creator3/1  "EPS_SteeringAngle_Flag"
  EPS_SteeringAngle/1 -> Bus Creator3/2  "EPS_SteeringAngle"
  EPS_Driver_Override/1 -> Bus Creator2/10  "EPS_Driver_Override"
  Bus Creator11/1 -> [Fusion_AdditionalInf]  "Fusion_AdditionalInf"
  Camera_Status/1 -> Bus Creator11/1  "Carema_Status"
  Sensor_Status/1 -> Bus Creator11/2  "Sensor_Status"
  Fusion_Status/1 -> Bus Creator11/3  "Fusion_Status"
  MP5_Work_State/1 -> Bus Creator/6  "MP5_Work_State"
  APA_AutoPark_WorkSt/1 -> Bus Creator/5  "APA_AutoPark_WorkSt"
  LDW_Warn_Mode/1 -> Bus Creator/4  "LDW_Warn_Mode"
  LkaFcnConf/1 -> Bus Creator/1  "LkaFcnConf"
  EPS_ESA_State/1 -> Bus Creator2/11  "EPS_ESA_State"
  ADIAve_g_ASWFaultStatus/1 -> Gain/1  "ADIAve_g_ASWFaultStatus"
  Gain/1 -> Terminator/1
  Gain1/1 -> Terminator1/1
  ADIAve_g_BSWFaultStatus/1 -> Gain1/1  "ADIAve_g_BSWFaultStatus"
  Gain2/1 -> Terminator2/1
  ADIAve_d_FuncFaultStatus/1 -> Gain2/1  "ADIAve_d_FuncFaultStatus"
  BCM_Double_Light_Switch/1 -> Bus Creator1/6  "BCM_Double_Light_Switch"
